simulink model "QPSK_map_demap_IQ"  (R2021a)
settings: Solver=VariableStepDiscrete  StartTime=0.0  StopTime=100/fs  RelTol=1e-3  EnableMultiTasking=on
PreLoadFcn:
  | %%%%%%%%%%%%%%%%%%%%%%%%%%%%%%%%%%%%%%%%%%%%%%%%%%%%%%%%%%%%%%%%%%%%%%%%%%%
  | % check to see if Simulink library folder is missing from the MATLAB path %
  | %%%%%%%%%%%%%%%%%%%%%%%%%%%%%%%%%%%%%%%%%%%%%%%%%%%%%%%%%%%%%%%%%%%%%%%%%%%
  | if isempty(strfind(path, 'rtlsdr_book_library'))
  | 
  |     % create error window
  |     fig_error = figure(...
  |         'Name', 'Error: RTL-SDR Book Library',...
  |         'Toolbar','none',...
  |         'MenuBar','none',...
  |         'NumberTitle','off',...
  |         'Resize','off',...
  |         'WindowStyle','modal');
  |     fig_error.Position(3) = 600;
  |     fig_error.Position(4) = 150;
  |     fig_axes = axes(...
  |         'Parent',fig_error,...
  |         'Position',[0,0,1,1],...
  |         'visible','off');
  |     % error message
  |     t_title = text(.05,.8,...
  |         'MISSING DIRECTORIES',...
  |         'FontSize',11.5);
  |     t_body = text(.075,.6,...
  |         [{'Simulink cannot find the  \it{<root>}\rm / \it{rtlsdr\_book\_library}\rm  folder in the \it{MATLAB Path}\rm.'},...
  |         {'Please set the MATLAB path following the instructions given in Exercise 2.4.'}],...
  |         'FontSize',10.5);
  |     % buttons
  |     btn_path = uicontrol(...
  |         'Parent',fig_error,...
  |         'String','Set Path Now',...
  |         'FontSize',10,...
  |         'Callback', 'pathtool; close(fig_error);',...
  |         'Position', [fig_error.Position(3)/2-210, 30, 200, 30]);
  |     btn_abort = uicontrol(...
  |         'Parent',fig_error,...
  |         'String','No thanks',...
  |         'FontSize',10,...
  |         'Callback', 'close(fig_error); abort=1;',...
  |         'Position', [fig_error.Position(3)/2+10, 30, 200, 30]);
  | 
  |     % pause to allow user to interact with error box
  |     uiwait(fig_error);
  | 
  |     % abort simulation
  |     try
  |         if abort==1
  |             set_param(gcs, 'SimulationCommand', 'stop');
  |         end
  |     end
  | 
  |     % if user has set path, allow diagram to be updated
  |     if ~exist('abort','var')
  |         % create error window
  |         fig_update = figure(...
  |             'Name', 'Update Diagram',...
  |             'Toolbar','none',...
  |             'MenuBar','none',...
  |             'NumberTitle','off',...
  |             'Resize','off');
  |         fig_update.Position(3) = 400;
  |         fig_update.Position(4) = 120;
  |         fig_axes = axes(...
  |             'Parent',fig_update,...
  |             'Position',[0,0,1,1],...
  |             'visible','off');
  |         % instruction message
  |         t_body = text(.075,.7,...
  |             'Once you have set the path, update the block diagram',...
  |             'FontSize',10.5);
  |         % button
  |         btn_update = uicontrol(...
  |             'Parent',fig_update,...
  |             'String','Update Block Diagram',...
  |             'FontSize',10,...
  |             'Callback', 'set_param(gcs,''SimulationCommand'',''update''); close(gcf)',...
  |             'Position', [fig_update.Position(3)/2-100, 30, 200, 30]);
  |     end
  | 
  |     % clear error components
  |     clear('fig_error','fig_update','fig_axes','t_title','t_body','btn_path','btn_abort','btn_update','abort');
  | 
  | end
  | %%%%%%%%%%%%%%%%%%%%%%%%%%%%%%%%%%%%%%%%%%%%%%%%%%%%%%%%%%%%%%%%%%%%%%%%%%%
  | 
  | MHz = 100;
  | fs = MHz * 1e6;
libraries: commdigbbndpm3 x2, commrandsrc3 x1, rtlsdr_book_library x1
CloseFcn:
  | closefcn_model;
Description:
  | Software, Simulation Examples and Design Exercises Licence Agreement
  | 
  | This license agreement refers to the simulation examples, design exercises and files,
  | and associated software MATLAB and Simulink resources that accompany the book:
  | 
  |      Title: Software Defined Radio using MATLAB & Simulink and the RTL-SDR
  |      Published by Strathclyde Academic Media, 2015
  |      Authored by Robert W. Stewart, Kenneth W. Barlee, Dale S.W. Atkinson,
  |      and Louise H. Crockett
  | 
  | and made available as a download from, www.desktopSDR.com or variously acquired
  | by other means such as via USB storage, cloud storage, disk or any other electronic
  | or optical or magnetic storage mechanism. These files and associated software may
  | be used subject to the terms of agreement of the conditions below:
  | 
  |     Copyright © 2015 Robert W. Stewart, Kenneth W. Barlee, Dale S.W. Atkinson,
  |     and Louise H. Crockett
  |     All rights reserved.
  | 
  | Redistribution and use in source and binary forms, with or without modification, are
  | permitted provided that the following conditions are met:
  | 
  |    1.  Redistributions of source code must retain the above copyright notice, this list of
  |         conditions and the following disclaimer.
  | 
  |    2.  Redistributions in binary form must reproduce the above copyright notice, this
  |         list of conditions and the following disclaimer in the documentation and/or other
  |         materials provided with the distribution.
  | 
  |    3.  Neither the name of the copyright holder nor the names of its contributors may
  |         be used to endorse or promote products derived from this software without
  |         specific prior written permission.
  | 
  |    4.  In all cases, the software is, and all modifications and derivatives of the
  |         software shall be, licensed to you solely for use in conjunction with The
  |         MathWorks, Inc. products and service offerings.
  | 
  | THIS SOFTWARE IS PROVIDED BY THE COPYRIGHT HOLDERS AND CONTRIBUTORS
  | "AS IS" AND ANY EXPRESS OR IMPLIED WARRANTIES, INCLUDING, BUT NOT LIMITED
  | TO, THE IMPLIED WARRANTIES OF MERCHANTABILITY AND FITNESS FOR A
  | PARTICULAR PURPOSE ARE DISCLAIMED. IN NO EVENT SHALL THE COPYRIGHT
  | HOLDER OR CONTRIBUTORS BE LIABLE FOR ANY DIRECT, INDIRECT, INCIDENTAL,
  | SPECIAL, EXEMPLARY, OR CONSEQUENTIAL DAMAGES (INCLUDING, BUT NOT
  | LIMITED TO, PROCUREMENT OF SUBSTITUTE GOODS OR SERVICES; LOSS OF USE,
  | DATA, OR PROFITS; OR BUSINESS INTERRUPTION) HOWEVER CAUSED AND ON ANY
  | THEORY OF LIABILITY, WHETHER IN CONTRACT, STRICT LIABILITY, OR TORT
  | (INCLUDING NEGLIGENCE OR OTHERWISE) ARISING IN ANY WAY OUT OF THE USE
  | OF THIS SOFTWARE, EVEN IF ADVISED OF THE POSSIBILITY OF SUCH DAMAGE.
  | 
  | 
  | Audio Tracks used in Simulations Examples and Design Exercises
  | 
  | The music and vocal files used within the Examples files and software within the book
  | were variously written, arranged, performed, recorded and produced by Garrey Rice,
  | Adam Struth, Jamie Struth, Iain Thistlethwaite and also Marshall Craigmyle who
  | collectively, and individually where appropriate, assert and retain all of their copyright,
  | performance and artistic rights. Permission to use and reproduce this music is
  | granted for all purposes associated with MATLAB and Simulink software and the
  | simulation examples and design exercises files that accompany this book. Requests to
  | use the music for any other purpose should be directed to: info@desktopSDR.com.
  | For information on music track names, full credits, and links to the musicians please
  | refer to www.desktopSDR.com/more/audio.
settings Model: Creator=desktopSDR Team  LastModifiedBy=Alex
settings SolverCC: AlgebraicLoopSolver=TrustRegion
settings DataIOCC: SaveFormat=Array  SaveOutput=off  SignalLogging=off  SaveTime=off  ReturnWorkspaceOutputs=off
settings OptimizationCC: BlockReduction=off  ConditionallyExecuteInputs=off  DefaultParameterBehavior=Inlined  LifeSpan=inf
settings DebuggingCC: AlgebraicLoopMsg=error  UnderspecifiedInitializationDetection=Classic  MergeDetectMultiDrivingBlocksExec=none  SolverPrmCheckMsg=warning  SFUnexpectedBacktrackingDiag=warning  SFNoUnconditionalDefaultTransitionDiag=warning  SFExecutionAtInitializationDiag=none  SFMachineParentedDataDiag=warning  ArithmeticOperatorsInVariantConditions=warning
settings HardwareCC: ProdBitPerPointer=32  ProdBitPerSizeT=32  ProdBitPerPtrDiffT=32  ProdLargestAtomicFloat=None  ProdIntDivRoundTo=Undefined  ProdEndianess=Unspecified  ProdWordSize=32  ProdHWDeviceType=ASIC/FPGA->ASIC/FPGA  ProdEqTarget=off
settings ModelReferenceCC: PropagateSignalLabelsOutOfModel=off
settings SFSimCC: SimUseLocalCustomCode=off  CustomCodeUndefinedFunction=UseInterfaceOnly
settings RTWCC: RTWUseLocalCustomCode=off
settings CodeAppCC: StateflowObjectComments=on
settings GRTTargetCC: TargetLangStandard=C89/C90 (ANSI)
settings ConfigComp: CovMetricSettings=dw  CovSaveCumulativeToWorkspaceVar=on  CovSaveSingleToWorkspaceVar=on  CovExternalEMLEnable=off  CovSFcnEnable=off

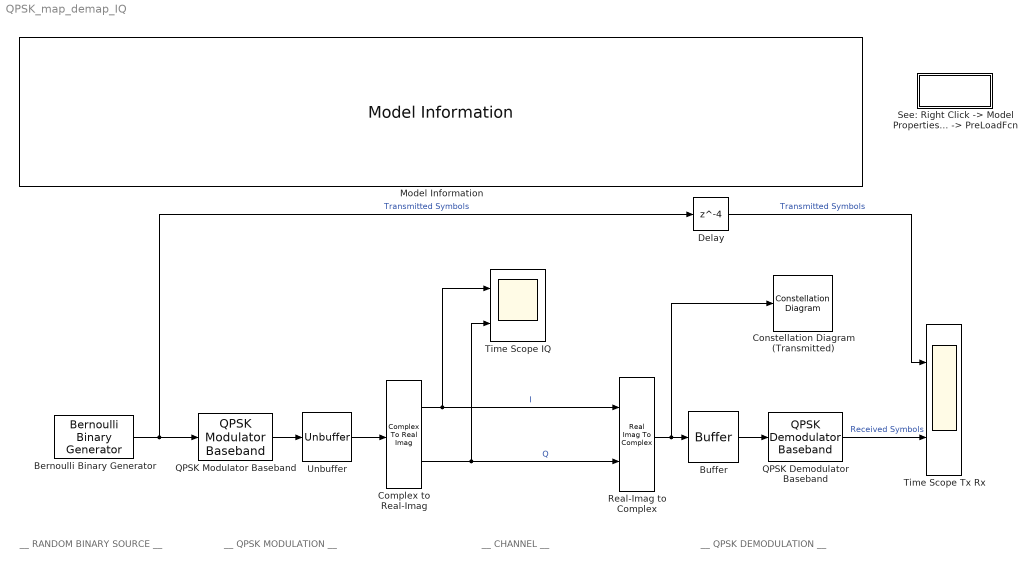
== system QPSK_map_demap_IQ ==
  note: __ RANDOM BINARY SOURCE __
  note: __ QPSK MODULATION __
  note: __ QPSK DEMODULATION __
  note: __ CHANNEL __
  Bernoulli Binary Generator : commrandsrc3/Bernoulli Binary Generator  ProbabilityOfZero=0.5  SeedSource=Parameter  Seed=61  SampleTime=1/fs  SamplesPerFrame=2  OutputDataType=boolean  SimulateUsing=Interpreted execution
  Buffer : Buffer  N=2
  Complex to Real-Imag : ComplexToRealImag
  Constellation Diagram (Transmitted) : ConstellationDiagram
  Delay : Delay  DelayLength=4  InputProcessing=Columns as channels (frame based)
  Model Information : rtlsdr_book_library/Additional Tools/Model Information/Model Information
      settings: SourceProductName=RTL-SDR Book Library
  QPSK Demodulator Baseband : commdigbbndpm3/QPSK Demodulator Baseband  OutType=Bit  DecType=Hard decision  VarSource=Dialog  Variance=1  Dec=Gray  Ph=pi/4  outDtype1=Inherit via internal rule  outDtype2=Inherit via internal rule  derotateFactorWordLen=16  derotateFactorDataTypeStr=Inherit: Same word length as input  derotateFactorLastDataTypeStr=Inherit: Same word length as input
  QPSK Modulator Baseband : commdigbbndpm3/QPSK Modulator Baseband  InType=Bit  Enc=Gray  Ph=pi/4  outDtype=double  outWordLen=16  outUDDataType=sfix(16)  outFracLenMode=User-defined  outFracLen=15  outDataTypeStr=double  outLastDataTypeStr=double
  Real-Imag to Complex : RealImagToComplex
  "See: Right Click -> Model Properties -> Callbacks -> PreLoadFcn " : Subsystem
      mask Display:
      | MHz = evalin('base', 'MHz');
      | fprintf(['fs = ',num2str(MHz),' MHz']);
  Time Scope Tx Rx : Scope  NumInputPorts=2
  Time Scope IQ : Scope  NumInputPorts=2
  Unbuffer : Unbuffer
  wires:
  Bernoulli Binary Generator/1 -> QPSK Modulator Baseband/1, Delay/1  "Transmitted Symbols"
  QPSK Demodulator Baseband/1 -> Time Scope Tx Rx/2  "Received Symbols"
  QPSK Modulator Baseband/1 -> Unbuffer/1
  Buffer/1 -> QPSK Demodulator Baseband/1
  Unbuffer/1 -> Complex to Real-Imag/1
  Real-Imag to Complex/1 -> Constellation Diagram (Transmitted)/1, Buffer/1
  Complex to Real-Imag/1 -> Time Scope IQ/1, Real-Imag to Complex/1  "I"
  Complex to Real-Imag/2 -> Time Scope IQ/2, Real-Imag to Complex/2  "Q"
  Delay/1 -> Time Scope Tx Rx/1  "Transmitted Symbols"

== system QPSK_map_demap_IQ/See: Right Click -> Model Properties -> Callbacks -> PreLoadFcn  ==
